simulink model "sepicmm_vs_sepicsm_noise"  (R2015a)
settings: Solver=ode45  StartTime=0.0  StopTime=0.05  RelTol=1e-3
values from neighbouring files (symbols this model uses):
  alpha = min(d1,d2)    [Final_2.m]    (also in Final_discreto.m)
  Ao = Aaum-L*Caum    [Final_2.m]
  Bo = [Baum L]    [Final_2.m]
  C1 = 190e-6    (= 0.00019)    [Final_2.m]    (also in Final_discreto.m = 0.0022)
  C2 = 190e-6    (= 0.00019)    [Final_2.m]    (also in Final_discreto.m = 0.0022)
  Co = [eye(size(Ao,1)-1) zeros(size(Ao,1)-1,1)]    [Final_2.m]
  Do = zeros(size(Ao,1)-1,2)    [Final_2.m]
  E0 = 20    [Final_2.m]    (also in Final_discreto.m = 36)
  ki = Ki_(5,1)    [Final_2.m]
  ks = [Ki_(1,1) Ki_(2,1) Ki_(3,1) Ki_(4,1) ]'    [Final_2.m]
  L1 = 2.3e-3    (= 0.0023)    [Final_2.m]    (also in Final_discreto.m = 0.00156)
  L2 = 330e-6    (= 0.00033)    [Final_2.m]    (also in Final_discreto.m = 0.00324)
  R0 = 44    [Final_2.m]    (also in Final_discreto.m = 50)
  R1 = 2.134    [Final_2.m]    (also in Final_discreto.m = 0.3)
  R2 = 0.234    [Final_2.m]    (also in Final_discreto.m = 0.3)
  V0 = 20    [Final_2.m]    (also in Final_discreto.m = 120)
libraries: powerlib x11, powerlib_meascontrol x1
settings Model: Creator=berme_000  LastModifiedBy=berme_000

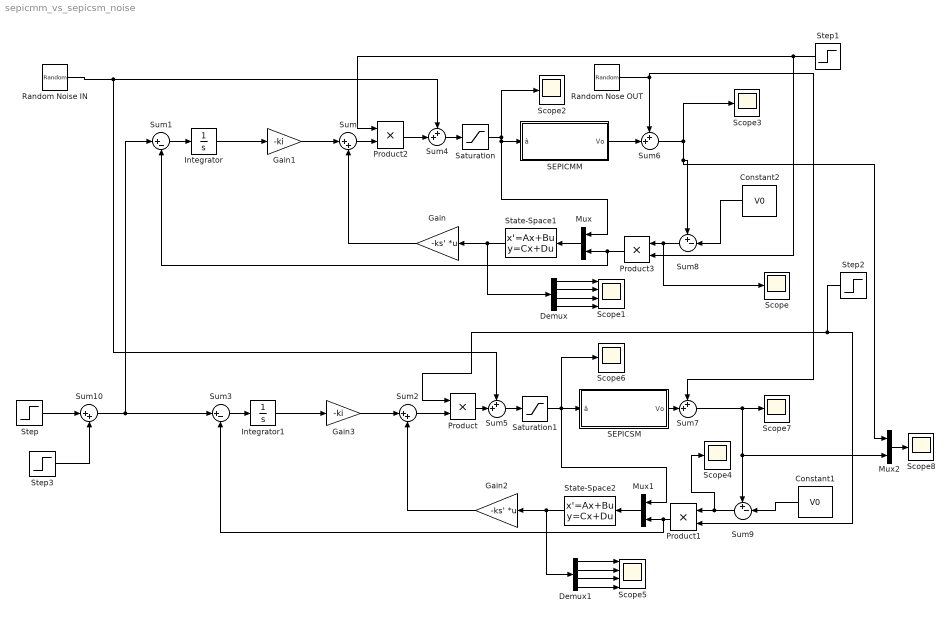
== system sepicmm_vs_sepicsm_noise ==
  Constant1 : Constant  Value=V0
  Constant2 : Constant  Value=V0
  Demux : Demux
  Demux1 : Demux
  Gain : Gain  Gain=-ks'  Multiplication=Matrix(K*u)
  Gain1 : Gain  Gain=-ki
  Gain2 : Gain  Gain=-ks'  Multiplication=Matrix(K*u)
  Gain3 : Gain  Gain=-ki
  Integrator : Integrator
  Integrator1 : Integrator
  Mux : Mux  Inputs=2
  Mux1 : Mux  Inputs=2
  Mux2 : Mux  Inputs=2
  Product{,1..3} (4 alike) : Product
  Random Noise IN : RandomNumber  Variance=.0001  SampleTime=0.0001
  Random Nose OUT : RandomNumber  Variance=0.001  SampleTime=0.0001
  "SEPICMM " : Subsystem
  "SEPICSM " : Subsystem
  Saturation : Saturate  UpperLimit=1-alpha  LowerLimit=0.5-alpha
  Saturation1 : Saturate  UpperLimit=1-alpha  LowerLimit=0.5-alpha
  Scope{,2..4,6..8} (7 alike) : Scope
      Scope settings: YMin=-120.8  YMax=-118.8
      Scope2 settings: YMin=0.216701  YMax=0.216701  SaveName=ScopeData3
      Scope3 settings: TimeRange=0.8  YMin=117  YMax=124.5  SaveName=ScopeData4
      Scope4 settings: YMin=-2.5  YMax=42.5  SaveName=ScopeData5
      Scope6 settings: YMin=-1  YMax=1  SaveName=ScopeData7
      Scope7 settings: TimeRange=1  YMin=52.525  YMax=52.95  SaveName=ScopeData8
      Scope8 settings: TimeRange=0.0005456720142856314  YMin=20.35  YMax=20.54  SaveName=output_sm_vs_mm
  Scope1 : Scope  NumInputPorts=4
      settings: YMin=-0.2~-0.35~-0.225~-0.5  YMax=0.9~0.05~0.025~5  SaveName=os_mm
  Scope5 : Scope  NumInputPorts=4
      settings: YMin=-50~-30~-10~-7  YMax=70~30~7.5~5  SaveName=os_sm
  State-Space1 : StateSpace  A=Ao  B=Bo  C=Co  D=Do  X0=0
  State-Space2 : StateSpace  A=Ao  B=Bo  C=Co  D=Do  X0=0
  Step : Step  Time=0.013  After=-1  SampleTime=0
  Step1 : Step  Time=0.008  SampleTime=0
  Step2 : Step  Time=0.008  SampleTime=0
  Step3 : Step  Time=0.02  After=5  SampleTime=0
  Sum : Sum  Inputs=|++
  Sum1 : Sum  Inputs=|+-
  Sum10 : Sum  Inputs=|++
  Sum2 : Sum  Inputs=|++
  Sum3 : Sum  Inputs=|+-
  Sum{4..7} (4 alike) : Sum  Inputs=++|
  Sum8 : Sum  Inputs=+-|
  Sum9 : Sum  Inputs=+-|
  wires:
  Mux/1 -> State-Space1/1
  State-Space1/1 -> Demux/1, Gain/1
  Integrator/1 -> Gain1/1
  Gain1/1 -> Sum/1
  Gain/1 -> Sum/2
  Sum6/1 -> Sum8/1, Mux2/1, Scope3/1
  Saturation/1 -> "SEPICMM "/1(â), Mux/1, Scope2/1
  Sum1/1 -> Integrator/1
  Mux1/1 -> State-Space2/1
  State-Space2/1 -> Demux1/1, Gain2/1
  Integrator1/1 -> Gain3/1
  Gain3/1 -> Sum2/1
  Gain2/1 -> Sum2/2
  Step2/1 -> Product/1, Product1/2
  Sum7/1 -> Sum9/1, Mux2/2, Scope7/1
  Saturation1/1 -> Scope6/1, Mux1/1, "SEPICSM "/1(â)
  Product1/1 -> Sum3/2, Mux1/2
  Sum10/1 -> Sum1/1, Sum3/1
  Sum3/1 -> Integrator1/1
  Mux2/1 -> Scope8/1
  Product3/1 -> Sum1/2, Mux/2
  Step1/1 -> Product2/1, Product3/2
  Random Noise IN/1 -> Sum4/1, Sum5/1
  Random Nose OUT/1 -> Sum7/1, Sum6/1
  "SEPICMM "/1(Vo) -> Sum6/2
  "SEPICSM "/1(Vo) -> Sum7/2
  Constant1/1 -> Sum9/2
  Sum9/1 -> Scope4/1, Product1/1
  Constant2/1 -> Sum8/2
  Sum8/1 -> Scope/1, Product3/1
  Product2/1 -> Sum4/2
  Sum4/1 -> Saturation/1
  Sum/1 -> Product2/2
  Product/1 -> Sum5/2
  Sum5/1 -> Saturation1/1
  Sum2/1 -> Product/2
  Demux/1 -> Scope1/1
  Demux/2 -> Scope1/2
  Demux/3 -> Scope1/3
  Demux/4 -> Scope1/4
  Demux1/1 -> Scope5/1
  Demux1/2 -> Scope5/2
  Demux1/3 -> Scope5/3
  Demux1/4 -> Scope5/4
  Step/1 -> Sum10/1
  Step3/1 -> Sum10/2

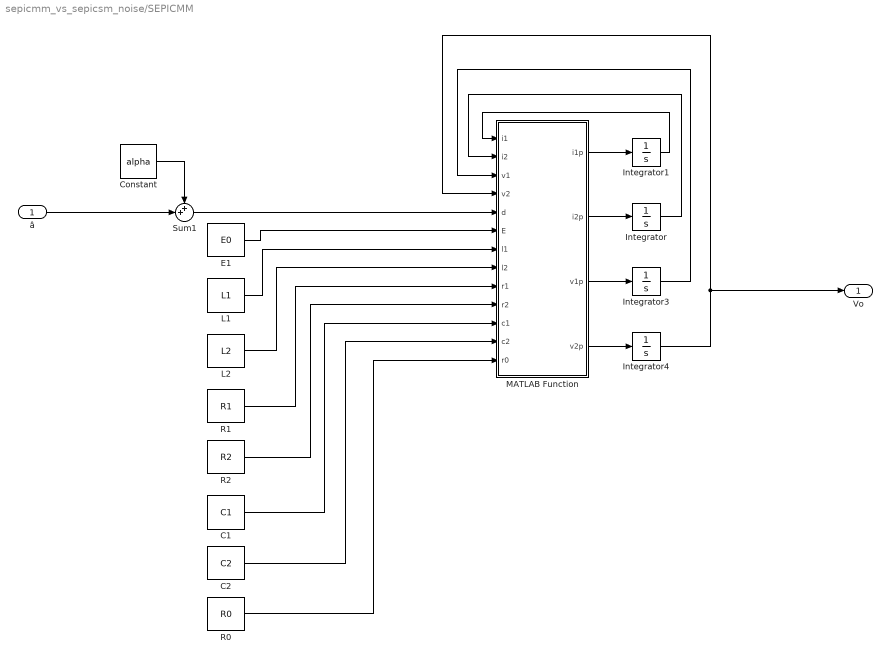
== system sepicmm_vs_sepicsm_noise/SEPICMM  ==
  â : Inport
  C1 : Constant  Value=C1
  C2 : Constant  Value=C2
  Constant : Constant  Value=alpha
  E1 : Constant  Value=E0
  Integrator{,1,3..4} (4 alike) : Integrator
  L1 : Constant  Value=L1
  L2 : Constant  Value=L2
  MATLAB Function : MATLAB Function  TreatAsAtomicUnit=on
  R0 : Constant  Value=R0
  R1 : Constant  Value=R1
  R2 : Constant  Value=R2
  Sum1 : Sum  Inputs=++|
  Vo : Outport
  wires:
  Constant/1 -> Sum1/1
  â/1 -> Sum1/2
  E1/1 -> MATLAB Function/6(E)
  Sum1/1 -> MATLAB Function/5(d)
  MATLAB Function/2(i2p) -> Integrator/1
  MATLAB Function/1(i1p) -> Integrator1/1
  MATLAB Function/3(v1p) -> Integrator3/1
  Integrator1/1 -> MATLAB Function/1(i1)
  Integrator/1 -> MATLAB Function/2(i2)
  Integrator3/1 -> MATLAB Function/3(v1)
  Integrator4/1 -> MATLAB Function/4(v2), Vo/1
  MATLAB Function/4(v2p) -> Integrator4/1
  L1/1 -> MATLAB Function/7(l1)
  L2/1 -> MATLAB Function/8(l2)
  R1/1 -> MATLAB Function/9(r1)
  R2/1 -> MATLAB Function/10(r2)
  C2/1 -> MATLAB Function/12(c2)
  C1/1 -> MATLAB Function/11(c1)
  R0/1 -> MATLAB Function/13(r0)

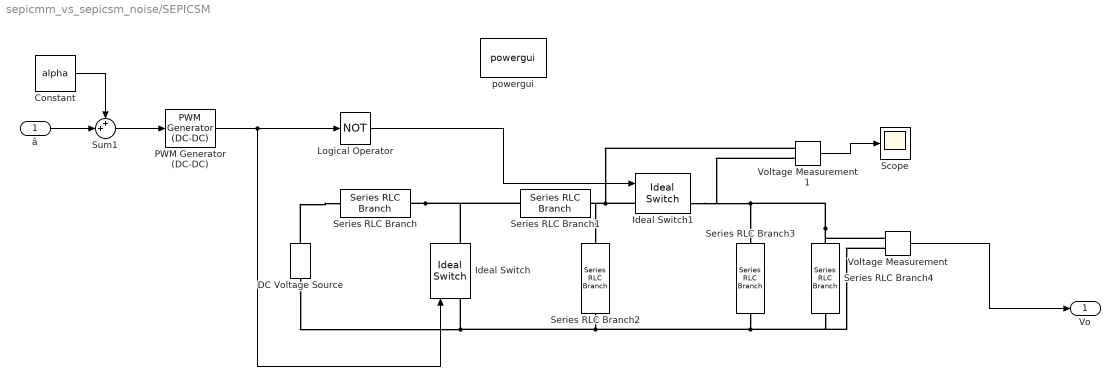
== system sepicmm_vs_sepicsm_noise/SEPICSM  ==
  â : Inport
  Constant : Constant  Value=alpha
  DC Voltage Source : powerlib/Electrical Sources/DC Voltage Source  Amplitude=E0  Measurements=None
  Ideal Switch : powerlib/Power Electronics/Ideal Switch  Ron=0.001  Lon=0  IC=0  Rs=1e5  Cs=inf  Measurements=on
  Ideal Switch1 : powerlib/Power Electronics/Ideal Switch  Ron=0.001  Lon=0  IC=0  Rs=1e5  Cs=inf  Measurements=on
  Logical Operator : Logic  Operator=NOT  AllPortsSameDT=off  OutDataTypeStr=boolean
  PWM Generator (DC-DC) : powerlib_meascontrol/Pulse & Signal Generators/PWM Generator (DC-DC)  Fsw=50000  Ts=0
  Scope : Scope
      settings: YMin=-9.23568e-13  YMax=-9.23568e-13  SaveName=ScopeData2
  Series RLC Branch : powerlib/Elements/Series RLC Branch  LConnTagsString=__new0  RConnTagsString=__new0  BranchType=RL  Resistance=R1  Inductance=L1  SetiL0=on  InitialCurrent=0  Capacitance=1e-6  Setx0=off  InitialVoltage=0  Measurements=None
  Series RLC Branch1 : powerlib/Elements/Series RLC Branch  LConnTagsString=__new0  RConnTagsString=__new0  BranchType=C  Resistance=1  Inductance=L1  SetiL0=off  InitialCurrent=0  Capacitance=C1  Setx0=on  InitialVoltage=0  Measurements=None
  Series RLC Branch2 : powerlib/Elements/Series RLC Branch  LConnTagsString=__new0  RConnTagsString=__new0  BranchType=RL  Resistance=R2  Inductance=L2  SetiL0=on  InitialCurrent=0  Capacitance=1e-6  Setx0=off  InitialVoltage=0  Measurements=None
  Series RLC Branch3 : powerlib/Elements/Series RLC Branch  LConnTagsString=__new0  RConnTagsString=__new0  BranchType=C  Resistance=1  Inductance=L1  SetiL0=off  InitialCurrent=0  Capacitance=C2  Setx0=on  InitialVoltage=0  Measurements=None
  Series RLC Branch4 : powerlib/Elements/Series RLC Branch  LConnTagsString=__new0  RConnTagsString=__new0  BranchType=R  Resistance=R0  Inductance=L1  SetiL0=off  InitialCurrent=0  Capacitance=1e-6  Setx0=off  InitialVoltage=0  Measurements=None
  Sum1 : Sum  Inputs=++|
  Voltage Measurement : powerlib/Measurements/Voltage Measurement  PhasorSimulation=off  OutputType=Complex  PSBequivalent=0
  Voltage Measurement1 : powerlib/Measurements/Voltage Measurement  PhasorSimulation=off  OutputType=Complex  PSBequivalent=0
  powergui : powerlib/powergui  Priority=1  SimulationMode=Continuous  SolverType=Tustin  SampleTime=50e-6  frequency=60  SPID=off  DisableSnubberDevices=off  DisableRonSwitches=off  DisableVfSwitches=off  SwTol=0  DisplayEquations=off  Interpol=off  methode=off  Ts=0  FunctionMessages=off  echomessages=off  HookPort=off  EnableUseOfTLC=off  x0status=blocks  frequencyindice=0  Pbase=100e6  ErrMax=1e-4  Iterations=50  UnitsV=kV  UnitsW=MW  buscounter=0  RestoreLinks=warning  ResistiveCurrentMeasurement=off  Frange=[0:2:500]  Ylog=off  Xlog=on  ShowGrid=off  save=off  variable=ZData  structure=0  ZoomFFT=off  StartTime=0.0  cycles=1  DisplayStyle=1  fundamental=60  FreqAxis=off  MaxFrequency=1000  frequencyindicesteady=1  RmsSteady=1  display=off
  Vo : Outport
  wires:
  â/1 -> Sum1/2
  Sum1/1 -> PWM Generator (DC-DC)/1
  Constant/1 -> Sum1/1
  PWM Generator (DC-DC)/1 -> Logical Operator/1, Ideal Switch/1
  Logical Operator/1 -> Ideal Switch1/1
  Voltage Measurement1/1 -> Scope/1
  Voltage Measurement/1 -> Vo/1
  connections:
  Series RLC Branch/RConn1 -- Series RLC Branch1/LConn1 -- Ideal Switch/RConn1
  Ideal Switch1/LConn1 -- Series RLC Branch1/RConn1 -- Series RLC Branch2/RConn1 -- Voltage Measurement1/LConn1
  Series RLC Branch2/LConn1 -- DC Voltage Source/LConn1 -- Ideal Switch/LConn1 -- Series RLC Branch3/RConn1 -- Voltage Measurement/LConn2 -- Series RLC Branch4/RConn1
  Voltage Measurement/LConn1 -- Series RLC Branch4/LConn1 -- Series RLC Branch3/LConn1 -- Ideal Switch1/RConn1 -- Voltage Measurement1/LConn2
  DC Voltage Source/RConn1 -- Series RLC Branch/LConn1

== matlab function sepicmm_vs_sepicsm_noise/SEPICMM /MATLAB Function ==
  data: i1 input; i2 input; v1 input; v2 input; i1p output; d input; E input; i2p output; v1p output; v2p output; l1 input; l2 input; r1 input; r2 input; c1 input; c2 input; r0 input
function [i1p,i2p,v1p,v2p]  = fcn(i1,i2,v1,v2,d,E,l1,l2,r1,r2,c1,c2,r0)
%#codegen
i1p=(E-i1*r1-(1-d)*(v1+v2))/l1;
i2p=(-v1*d+(1-d)*v2-i2*r2)/l2;
v1p=(i2*d+i1*(1-d))/c1;
v2p=(-v2/r0+(1-d)*(i1-i2))/c2;
